simulink model "FlightDynamicModelBlackOut"  (R2017a)
settings: Solver=VariableStepAuto  StartTime=0.0  StopTime=200  RelTol=1e-3
undefined symbols (not defined in the file or in its folder): F, Light, MIL
libraries: simulink x13, aerolibatmos2 x1, aerolibwind2 x1
settings Model: Creator=740582  LastModifiedBy=740582
settings OptimizationCC: LifeSpan=inf
settings DebuggingCC: SFExecutionAtInitializationDiag=none

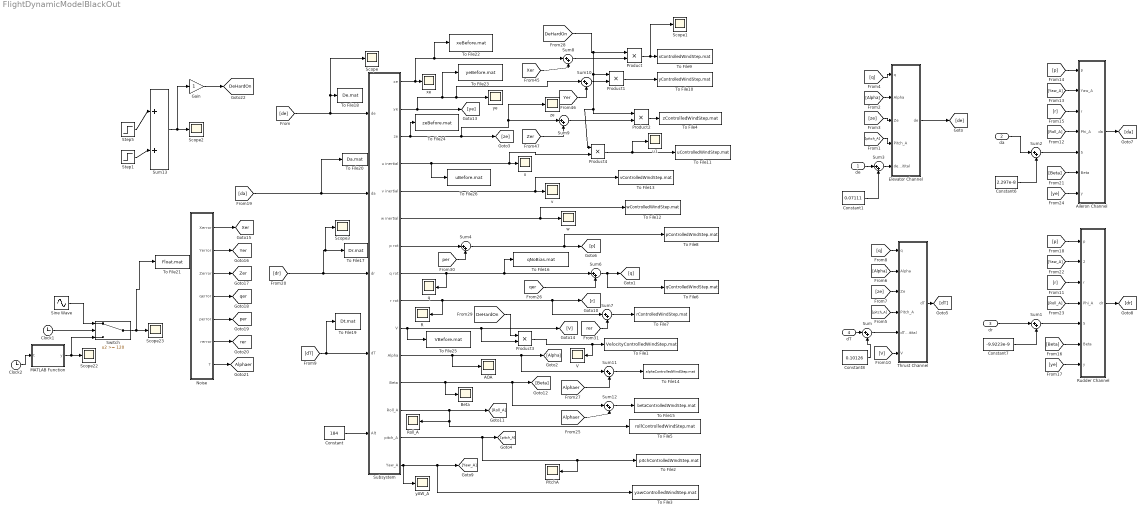
== system FlightDynamicModelBlackOut ==
  de : Inport
  da : Inport  Port=2
  dr : Inport  Port=3
  dT : Inport  Port=4
  AOA : Scope
  Aileron Channel : Subsystem
  "Beta " : Scope
  Clock1 : Clock
  Clock2 : Clock
  Constant : Constant  Value=184
  Constant1 : Constant  Value=0.07111
  Constant6 : Constant  Value=2.297e-8
  Constant7 : Constant  Value=-9.9223e-9
  Constant8 : Constant  Value=0.10126
  Elevator Channel : Subsystem
  Gain : Gain
  MATLAB Function : MATLAB Function  TreatAsAtomicUnit=on
  Noise : Subsystem
  PitchA : Scope
  Product{,1..4} (5 alike) : Product
  "R " : Scope
  "Roll_A " : Scope
  Rudder Channel : Subsystem
  Scope{,1..3,22..23} (6 alike) : Scope
  Sine Wave : Sin  Amplitude=0.1745  Frequency=0.1833  Phase=pi  SampleTime=0
  Step1 : Step  Time=80  SampleTime=20
  Step5 : Step  Time=40  Before=1  After=0  SampleTime=20
  Subsystem : Subsystem
  Sum{,1..4,6..13} (13 alike) : Sum  Inputs=|++
  Switch : Switch  Threshold=120
  Thrust Channel : Subsystem
  To File1 : ToFile  Filename=VelocityControlledWindStep.mat  MatrixName=VelocityControlledWindStep
  To File10 : ToFile  Filename=yControlledWindStep.mat  MatrixName=yControlledWindStep
  To File11 : ToFile  Filename=uControlledWindStep.mat  MatrixName=uControlledWindStep
  To File12 : ToFile  Filename=wControlledWindStep.mat  MatrixName=wControlledWindStep
  To File13 : ToFile  Filename=vControlledWindStep.mat  MatrixName=vControlledWindStep
  To File14 : ToFile  Filename=alphaControlledWindStep.mat  MatrixName=alphaControlledWindStep
  To File15 : ToFile  Filename=betaControlledWindStep.mat  MatrixName=betaControlledWindStep
  To File16 : ToFile  Filename=qNoBias.mat  MatrixName=qNoBias
  To File17 : ToFile  Filename=Dr.mat  MatrixName=Dr
  To File18 : ToFile  Filename=De.mat  MatrixName=De
  To File19 : ToFile  Filename=Dt.mat  MatrixName=Dt
  To File2 : ToFile  Filename=pitchControlledWindStep.mat  MatrixName=pitchControlledWindStep
  To File20 : ToFile  Filename=Da.mat  MatrixName=Da
  To File21 : ToFile  Filename=Float.mat  MatrixName=Float
  To File22 : ToFile  Filename=xeBefore.mat  MatrixName=xeBefore
  To File23 : ToFile  Filename=yeBefore.mat  MatrixName=yeBefore
  To File24 : ToFile  Filename=zeBefore.mat  MatrixName=zeBefore
  To File25 : ToFile  Filename=VBefore.mat  MatrixName=VBefore
  To File26 : ToFile  Filename=uBefore.mat  MatrixName=uBefore
  To File3 : ToFile  Filename=yawControlledWindStep.mat  MatrixName=yawControlledWindStep
  To File4 : ToFile  Filename=zControlledWindStep.mat  MatrixName=zControlledWindStep
  To File5 : ToFile  Filename=rollControlledWindStep.mat  MatrixName=rollControlledWindStep
  To File6 : ToFile  Filename=qControlledWindStep.mat  MatrixName=qControlledWindStep
  To File7 : ToFile  Filename=rControlledWindStep.mat  MatrixName=rControlledWindStep
  To File8 : ToFile  Filename=pControlledWindStep.mat  MatrixName=pControlledWindStep
  To File9 : ToFile  Filename=xControlledWindStep.mat  MatrixName=xControlledWindStep
  V : Scope
  q : Scope
  u : Scope
  u1 : Scope
  v : Scope
  w : Scope
  xe : Scope
  yAW_A : Scope
  ye : Scope
  ze : Scope
  tag scope: Alphaer=global, DeHardOn=global, Xer=global, Yer=global, Zer=global, per=global, qer=global, rer=global
  wires:
  Sum1/1 -> Rudder Channel/5(dr_Initital)
  [ze] -> Thrust Channel/3(Ze)
  [p] -> Rudder Channel/1(p)
  [r] -> Aileron Channel/3(r)
  [Beta] -> Rudder Channel/6(Beta)
  [V] -> Thrust Channel/6(V)
  [p] -> Aileron Channel/1(p)
  [pitch_A] -> Elevator Channel/4(Pitch_A)
  Sum3/1 -> Elevator Channel/5(de_Initital)
  Thrust Channel/1(dT) -> [dT]
  Rudder Channel/1(dr) -> [dr]
  [Roll_A] -> Aileron Channel/4(Phi_A)
  [Beta] -> Aileron Channel/6(Beta)
  [Alpha] -> Elevator Channel/2(Alpha)
  [r] -> Rudder Channel/3(r)
  dT/1 -> Sum/1
  [ze] -> Elevator Channel/3(Ze)
  [ye] -> Aileron Channel/7(y)
  da/1 -> Sum2/1
  Sum2/1 -> Aileron Channel/5(da_Initital)
  [q] -> Elevator Channel/1(q)
  [pitch_A] -> Thrust Channel/4(Pitch_A)
  [Yaw_A] -> Aileron Channel/2(Yaw_A)
  [ye] -> Rudder Channel/7(y)
  [Yaw_A] -> Rudder Channel/2(Yaw_A)
  Aileron Channel/1(da) -> [da]
  de/1 -> Sum3/1
  Elevator Channel/1(de) -> [de]
  [Roll_A] -> Rudder Channel/4(Phi_A)
  [q] -> Thrust Channel/1(q)
  Sum/1 -> Thrust Channel/5(dT_Initital)
  [Alpha] -> Thrust Channel/2(Alpha)
  dr/1 -> Sum1/1
  Subsystem/13(Roll_A) -> To File5/1, "Roll_A "/1, [Roll_A]
  Subsystem/15(Yaw_A) -> yAW_A/1, To File3/1, [Yaw_A]
  Subsystem/14(pitch_A) -> PitchA/1, To File2/1, [pitch_A]
  Subsystem/10(V) -> To File25/1, Product3/2, [V]
  Subsystem/6(w inertial) -> w/1, To File12/1
  Subsystem/5(v inertial) -> To File13/1, v/1
  Constant1/1 -> Sum3/2
  Constant/1 -> Subsystem/5(Alt)
  Constant6/1 -> Sum2/2
  Constant8/1 -> Sum/2
  Constant7/1 -> Sum1/2
  Subsystem/1(xe) -> To File22/1, Sum8/1, xe/1
  Subsystem/3(ze) -> To File24/1, ze/1, Sum9/1, [ze]
  Subsystem/2(ye) -> [ye], To File23/1, Sum10/1, ye/1
  Subsystem/8(q rot) -> q/1, Sum6/1, To File16/1
  Subsystem/4(u inertial) -> To File26/1, Product4/2, u/1
  Subsystem/11(Alpha) -> AOA/1, Sum11/1, [Alpha]
  Subsystem/12(Beta) -> Sum12/1, [Beta], "Beta "/1
  Noise/7(Alphaerror) -> [Alphaer]
  Noise/1(Xerror) -> [Xer]
  Noise/2(Yerror) -> [Yer]
  Noise/3(Zerror) -> [Zer]
  Noise/4(qerror) -> [qer]
  Noise/5(perror) -> [per]
  Noise/6(rerror) -> [rer]
  [rer] -> Sum7/2
  [per] -> Sum4/2
  Sum7/1 -> To File7/1
  Subsystem/9(r rot) -> "R "/1, Sum7/1, [r]
  [Yer] -> Sum10/2
  [Xer] -> Sum8/2
  [Zer] -> Sum9/2
  [Alphaer] -> Sum12/2
  [Alphaer] -> Sum11/2
  Sum11/1 -> To File14/1
  Sum12/1 -> To File15/1
  Subsystem/7(p rot) -> Sum4/1
  Sum4/1 -> To File8/1, [p]
  Sum6/1 -> To File6/1, [q]
  [qer] -> Sum6/2
  [DeHardOn] -> Product/1, Product1/1, Product4/1, Product2/1
  [dT] -> To File19/1, Subsystem/4(dT)
  Switch/1 -> To File21/1, Scope23/1
  Clock1/1 -> Switch/2
  Sine Wave/1 -> Switch/1
  Clock2/1 -> MATLAB Function/1(t)
  MATLAB Function/1(y) -> Scope22/1, Switch/3
  [dr] -> Scope3/1, To File17/1, Subsystem/3(dr)
  [da] -> To File20/1, Subsystem/2(da)
  [de] -> Scope/1, To File18/1, Subsystem/1(de)
  Step1/1 -> Sum13/2
  Step5/1 -> Sum13/1
  Sum13/1 -> Gain/1, Scope2/1
  Sum8/1 -> Product/2
  Product/1 -> Scope1/1, To File9/1
  Sum10/1 -> Product1/2
  Product1/1 -> To File10/1
  Sum9/1 -> Product2/2
  Product2/1 -> To File4/1
  Product3/1 -> V/1, To File1/1
  [DeHardOn] -> Product3/1
  Product4/1 -> u1/1, To File11/1
  Gain/1 -> [DeHardOn]

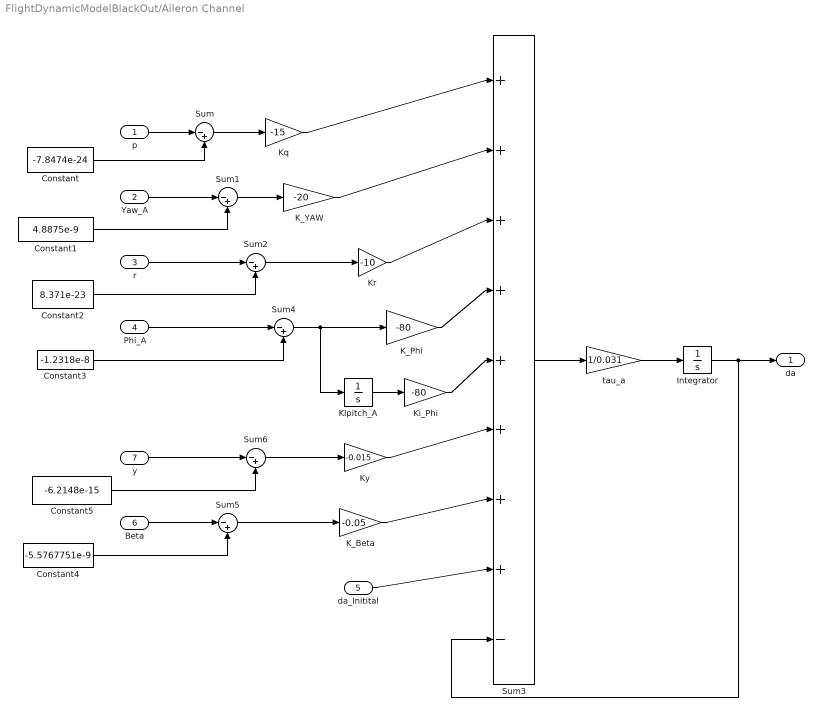
== system FlightDynamicModelBlackOut/Aileron Channel ==
  p : Inport
  Yaw_A : Inport  Port=2
  r : Inport  Port=3
  Phi_A : Inport  Port=4
  da_Initital : Inport  Port=5
  Beta : Inport  Port=6
  y : Inport  Port=7
  Constant : Constant  Value=-7.8474e-24
  Constant1 : Constant  Value=4.8875e-9
  Constant2 : Constant  Value=8.371e-23
  Constant3 : Constant  Value=-1.2318e-8
  Constant4 : Constant  Value=-5.5767751e-9
  Constant5 : Constant  Value=-6.2148e-15
  Integrator : Integrator  InitialCondition=2.297e-8  LimitOutput=on  UpperSaturationLimit=0.3490658504  LowerSaturationLimit=-0.3490658504
  KIpitch_A : Integrator
  K_Beta : Gain  Gain=-0.05
  K_Phi : Gain  Gain=-80
  K_YAW : Gain  Gain=-20
  Ki_Phi : Gain  Gain=-80
  Kq : Gain  Gain=-15
  Kr : Gain  Gain=-10
  Ky : Gain  Gain=-0.015
  Sum{,1..2,4..6} (6 alike) : Sum  Inputs=|-+
  Sum3 : Sum  Inputs=|++++++++-
  tau_a : Gain  Gain=1/0.031
  da : Outport  OutMin=[-0.3490658504]  OutMax=[0.3490658504]
  wires:
  Constant/1 -> Sum/2
  p/1 -> Sum/1
  Yaw_A/1 -> Sum1/1
  r/1 -> Sum2/1
  Phi_A/1 -> Sum4/1
  Constant1/1 -> Sum1/2
  Constant2/1 -> Sum2/2
  Constant3/1 -> Sum4/2
  Sum/1 -> Kq/1
  Sum1/1 -> K_YAW/1
  Sum2/1 -> Kr/1
  Sum4/1 -> KIpitch_A/1, K_Phi/1
  Kq/1 -> Sum3/1
  K_YAW/1 -> Sum3/2
  Kr/1 -> Sum3/3
  K_Phi/1 -> Sum3/4
  Sum3/1 -> tau_a/1
  Ki_Phi/1 -> Sum3/5
  KIpitch_A/1 -> Ki_Phi/1
  tau_a/1 -> Integrator/1
  Integrator/1 -> Sum3/9, da/1
  da_Initital/1 -> Sum3/8
  K_Beta/1 -> Sum3/7
  Beta/1 -> Sum5/1
  Sum5/1 -> K_Beta/1
  Constant4/1 -> Sum5/2
  Ky/1 -> Sum3/6
  y/1 -> Sum6/1
  Sum6/1 -> Ky/1
  Constant5/1 -> Sum6/2

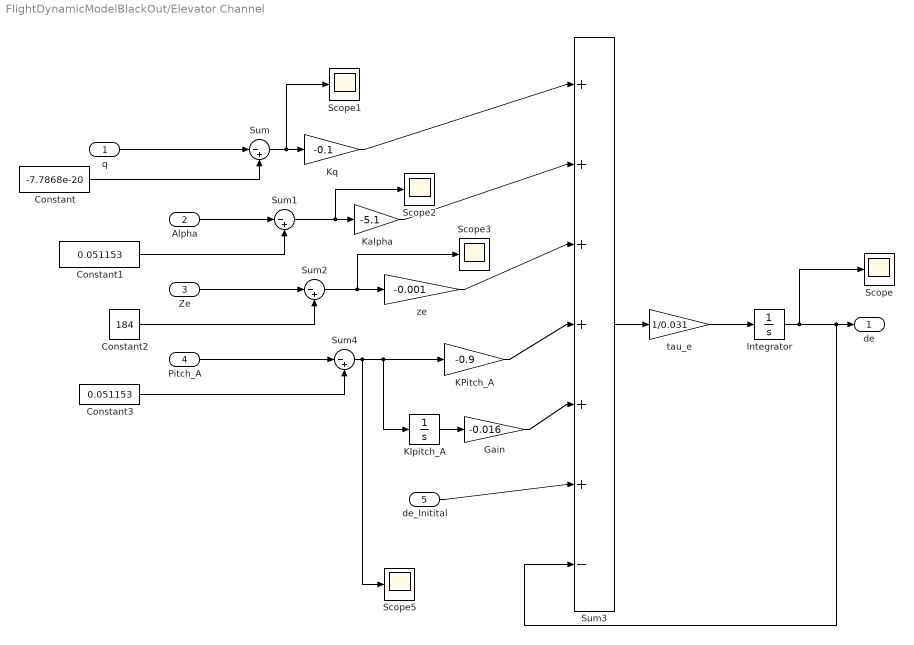
== system FlightDynamicModelBlackOut/Elevator Channel ==
  q : Inport
  Alpha : Inport  Port=2
  Ze : Inport  Port=3
  Pitch_A : Inport  Port=4
  de_Initital : Inport  Port=5
  Constant : Constant  Value=-7.7868e-20
  Constant1 : Constant  Value=0.051153
  Constant2 : Constant  Value=184
  Constant3 : Constant  Value=0.051153
  Gain : Gain  Gain=-0.016
  Integrator : Integrator  InitialCondition=0.07111  LimitOutput=on  UpperSaturationLimit=0.3490658504  LowerSaturationLimit=-0.6981317008
  KIpitch_A : Integrator
  KPitch_A : Gain  Gain=-0.9
  Kalpha : Gain  Gain=-5.1
  Kq : Gain  Gain=-0.1
  Scope{,1..3,5} (5 alike) : Scope
  Sum{,1..2,4} (4 alike) : Sum  Inputs=|-+
  Sum3 : Sum  Inputs=|++++++-
  tau_e : Gain  Gain=1/0.031
  ze : Gain  Gain=-0.001
  de : Outport  OutMin=[-0.6981317008504]  OutMax=[0.3490658504]
  wires:
  Alpha/1 -> Sum1/1
  Ze/1 -> Sum2/1
  Pitch_A/1 -> Sum4/1
  Constant1/1 -> Sum1/2
  Constant2/1 -> Sum2/2
  Constant3/1 -> Sum4/2
  Sum/1 -> Scope1/1, Kq/1
  Sum1/1 -> Scope2/1, Kalpha/1
  Sum2/1 -> Scope3/1, ze/1
  Sum4/1 -> Scope5/1, KIpitch_A/1, KPitch_A/1
  Kq/1 -> Sum3/1
  Kalpha/1 -> Sum3/2
  ze/1 -> Sum3/3
  KPitch_A/1 -> Sum3/4
  Sum3/1 -> tau_e/1
  de_Initital/1 -> Sum3/6
  Gain/1 -> Sum3/5
  KIpitch_A/1 -> Gain/1
  tau_e/1 -> Integrator/1
  Integrator/1 -> Scope/1, Sum3/7, de/1
  q/1 -> Sum/1
  Constant/1 -> Sum/2

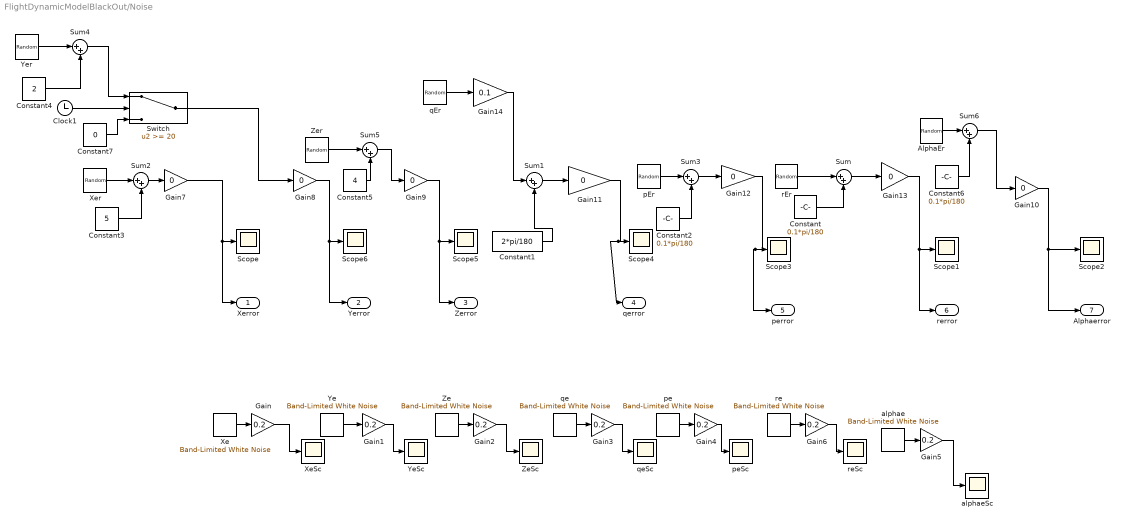
== system FlightDynamicModelBlackOut/Noise ==
  AlphaEr : UniformRandomNumber  Minimum=-0.001*0.1014*pi/180  Maximum=0.001*0.1014*pi/180  SampleTime=0.1
  Clock1 : Clock
  Constant : Constant  Value=0.1*pi/180
  Constant1 : Constant  Value=2*pi/180
  Constant2 : Constant  Value=0.1*pi/180
  Constant3 : Constant  Value=5
  Constant4 : Constant  Value=2
  Constant5 : Constant  Value=4
  Constant6 : Constant  Value=0.1*pi/180
  Constant7 : Constant  Value=0
  Gain{,1..6} (7 alike) : Gain  Gain=0.2
  Gain{7..13} (7 alike) : Gain  Gain=0
  Gain14 : Gain  Gain=0.1
  Scope{,1..6} (7 alike) : Scope
  Sum{,1..6} (7 alike) : Sum  Inputs=|++
  Switch : Switch  Threshold=20
  Xe : simulink/Sources/Band-Limited White Noise  Cov=[0.8]  Ts=0.1  seed=[23341]
  XeSc : Scope
  Xer : UniformRandomNumber  Minimum=-2  Maximum=2  SampleTime=0.1
  Ye : simulink/Sources/Band-Limited White Noise  Cov=[0.1*0.5]  Ts=0.1  seed=[23341]
  YeSc : Scope
  Yer : UniformRandomNumber  Minimum=-0.05  Maximum=0.05  SampleTime=0.1
  Ze : simulink/Sources/Band-Limited White Noise  Cov=[0.1]  Ts=0.1  seed=[23341]
  ZeSc : Scope
  Zer : UniformRandomNumber  SampleTime=0.1
  alphae : simulink/Sources/Band-Limited White Noise  Cov=[0.0000008]  Ts=0.1  seed=[23341]
  alphaeSc : Scope
  pEr : UniformRandomNumber  Minimum=-0.001*1.8707*pi/180  Maximum=0.001*1.8707*pi/180  SampleTime=0.1
  pe : simulink/Sources/Band-Limited White Noise  Cov=[0.0001]  Ts=0.1  seed=[23341]
  peSc : Scope
  qEr : UniformRandomNumber  Minimum=-0.001*1.8707*pi/180  Maximum=0.001*1.8707*pi/180  SampleTime=0.1
  qe : simulink/Sources/Band-Limited White Noise  Cov=[0.0001]  Ts=0.1  seed=[23341]
  qeSc : Scope
  rEr : UniformRandomNumber  Minimum=-0.001*1.8707*pi/180  Maximum=0.001*1.8707*pi/180  SampleTime=0.1
  re : simulink/Sources/Band-Limited White Noise  Cov=[0.0001]  Ts=0.1  seed=[23341]
  reSc : Scope
  Xerror : Outport
  Yerror : Outport  Port=2
  Zerror : Outport  Port=3
  qerror : Outport  Port=4
  perror : Outport  Port=5
  rerror : Outport  Port=6
  Alphaerror : Outport  Port=7
  wires:
  alphae/1 -> Gain5/1
  re/1 -> Gain6/1
  Ze/1 -> Gain2/1
  Ye/1 -> Gain1/1
  pe/1 -> Gain4/1
  Xe/1 -> Gain/1
  qe/1 -> Gain3/1
  Gain/1 -> XeSc/1
  Gain1/1 -> YeSc/1
  Gain2/1 -> ZeSc/1
  Gain3/1 -> qeSc/1
  Gain4/1 -> peSc/1
  Gain6/1 -> reSc/1
  Gain5/1 -> alphaeSc/1
  Gain7/1 -> Xerror/1, Scope/1
  Gain8/1 -> Yerror/1, Scope6/1
  Gain9/1 -> Zerror/1, Scope5/1
  Gain10/1 -> Alphaerror/1, Scope2/1
  Gain13/1 -> rerror/1, Scope1/1
  Gain12/1 -> perror/1, Scope3/1
  Gain11/1 -> qerror/1, Scope4/1
  Sum1/1 -> Gain11/1
  Sum3/1 -> Gain12/1
  pEr/1 -> Sum3/1
  rEr/1 -> Sum/1
  Sum/1 -> Gain13/1
  Sum2/1 -> Gain7/1
  Constant/1 -> Sum/2
  Constant2/1 -> Sum3/2
  Constant1/1 -> Sum1/2
  Xer/1 -> Sum2/1
  Yer/1 -> Sum4/1
  qEr/1 -> Gain14/1
  AlphaEr/1 -> Sum6/1
  Sum6/1 -> Gain10/1
  Constant3/1 -> Sum2/2
  Constant4/1 -> Sum4/2
  Constant6/1 -> Sum6/2
  Constant7/1 -> Switch/3
  Clock1/1 -> Switch/2
  Zer/1 -> Sum5/1
  Sum5/1 -> Gain9/1
  Constant5/1 -> Sum5/2
  Sum4/1 -> Switch/1
  Switch/1 -> Gain8/1
  Gain14/1 -> Sum1/1

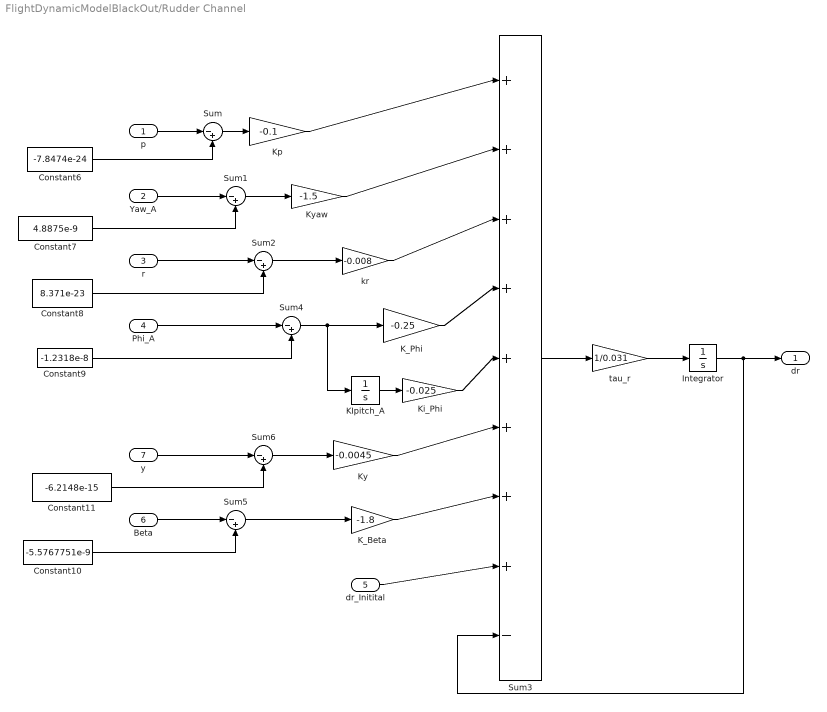
== system FlightDynamicModelBlackOut/Rudder Channel ==
  p : Inport
  Yaw_A : Inport  Port=2
  r : Inport  Port=3
  Phi_A : Inport  Port=4
  dr_Initital : Inport  Port=5
  Beta : Inport  Port=6
  y : Inport  Port=7
  Constant10 : Constant  Value=-5.5767751e-9
  Constant11 : Constant  Value=-6.2148e-15
  Constant6 : Constant  Value=-7.8474e-24
  Constant7 : Constant  Value=4.8875e-9
  Constant8 : Constant  Value=8.371e-23
  Constant9 : Constant  Value=-1.2318e-8
  Integrator : Integrator  InitialCondition=-9.9223e-9  LimitOutput=on  UpperSaturationLimit=0.5235987756  LowerSaturationLimit=-0.5235987756
  KIpitch_A : Integrator
  K_Beta : Gain  Gain=-1.8
  K_Phi : Gain  Gain=-0.25
  Ki_Phi : Gain  Gain=-0.025
  Kp : Gain  Gain=-0.1
  Ky : Gain  Gain=-0.0045
  Kyaw : Gain  Gain=-1.5
  Sum{,1..2,4..6} (6 alike) : Sum  Inputs=|-+
  Sum3 : Sum  Inputs=|++++++++-
  "kr " : Gain  Gain=-0.008
  tau_r : Gain  Gain=1/0.031
  dr : Outport  OutMin=[-0.5235987756]  OutMax=[0.5235987756]
  wires:
  dr_Initital/1 -> Sum3/8
  Sum6/1 -> Ky/1
  y/1 -> Sum6/1
  Beta/1 -> Sum5/1
  Sum5/1 -> K_Beta/1
  Constant10/1 -> Sum5/2
  K_Beta/1 -> Sum3/7
  Phi_A/1 -> Sum4/1
  Constant7/1 -> Sum1/2
  Ki_Phi/1 -> Sum3/5
  Constant11/1 -> Sum6/2
  K_Phi/1 -> Sum3/4
  Constant6/1 -> Sum/2
  Sum1/1 -> Kyaw/1
  Kyaw/1 -> Sum3/2
  KIpitch_A/1 -> Ki_Phi/1
  Yaw_A/1 -> Sum1/1
  Sum/1 -> Kp/1
  "kr "/1 -> Sum3/3
  r/1 -> Sum2/1
  Sum3/1 -> tau_r/1
  Sum2/1 -> "kr "/1
  Integrator/1 -> Sum3/9, dr/1
  Sum4/1 -> K_Phi/1, KIpitch_A/1
  tau_r/1 -> Integrator/1
  Kp/1 -> Sum3/1
  Constant8/1 -> Sum2/2
  Ky/1 -> Sum3/6
  p/1 -> Sum/1
  Constant9/1 -> Sum4/2

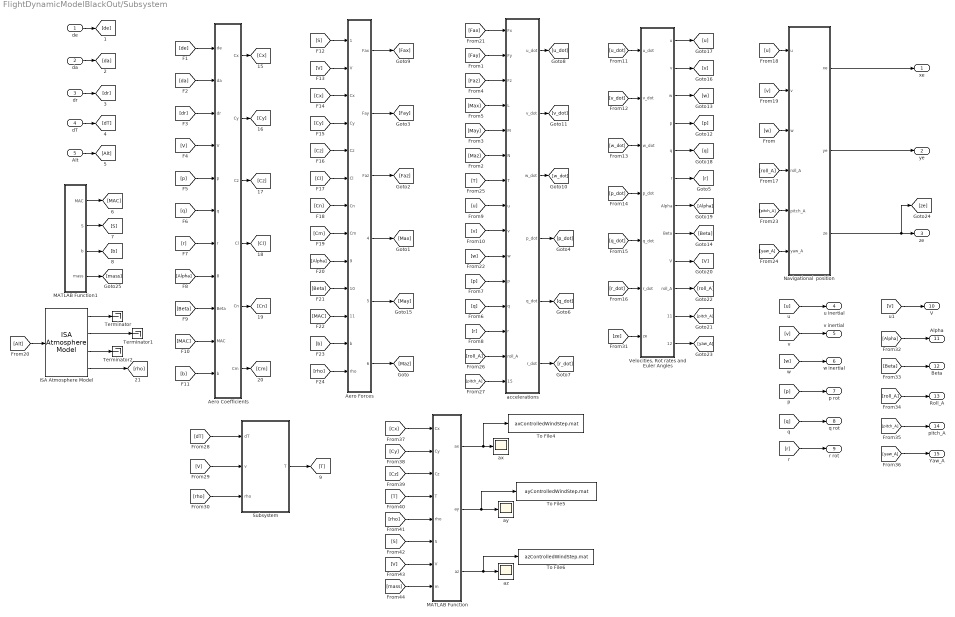
== system FlightDynamicModelBlackOut/Subsystem ==
  de : Inport
  da : Inport  Port=2
  dr : Inport  Port=3
  dT : Inport  Port=4
  Alt : Inport  Port=5
  Aero Coefficients : MATLAB Function  TreatAsAtomicUnit=on
  Aero Forces : MATLAB Function  TreatAsAtomicUnit=on
  ISA Atmosphere Model : aerolibatmos2/ISA Atmosphere Model  custom=off  g=9.80665  gamma=1.4  R=287.0531  L=0.0065  h_trop=11000  h_strat=20000  rho0=1.225  P0=101325  T0=288.15  h0=0
      settings: SourceProductName=Aerospace Blockset
  MATLAB Function : MATLAB Function  TreatAsAtomicUnit=on
  MATLAB Function1 : MATLAB Function  TreatAsAtomicUnit=on
  Navigational  position : Subsystem
  Subsystem : Subsystem
  Terminator : Terminator
  Terminator1 : Terminator
  Terminator2 : Terminator
  To File4 : ToFile  Filename=axControlledWindStep.mat  MatrixName=axControlledWindStep
  To File5 : ToFile  Filename=ayControlledWindStep.mat  MatrixName=ayControlledWindStep
  To File6 : ToFile  Filename=azControlledWindStep.mat  MatrixName=azControlledWindStep
  "Velocities, Rot rates and Euler Angles" : Subsystem
  accelerations : MATLAB Function  TreatAsAtomicUnit=on
  ax : Scope
  ay : Scope
  az : Scope
  xe : Outport
  ye : Outport  Port=2
  ze : Outport  Port=3
  u inertial : Outport  Port=4
  v inertial : Outport  Port=5
  w inertial : Outport  Port=6
  p rot : Outport  Port=7
  q rot : Outport  Port=8
  r rot : Outport  Port=9
  V : Outport  Port=10
  Alpha : Outport  Port=11
  Beta : Outport  Port=12
  Roll_A : Outport  Port=13
  pitch_A : Outport  Port=14
  Yaw_A : Outport  Port=15
  wires:
  de/1 -> [de]
  da/1 -> [da]
  dr/1 -> [dr]
  dT/1 -> [dT]
  Alt/1 -> [Alt]
  MATLAB Function1/1(MAC) -> [MAC]
  MATLAB Function1/2(S) -> [S]
  MATLAB Function1/3(b) -> [b]
  [de] -> Aero Coefficients/1(de)
  [da] -> Aero Coefficients/2(da)
  [dr] -> Aero Coefficients/3(dr)
  [V] -> Aero Coefficients/4(V)
  [b] -> Aero Coefficients/11(b)
  [MAC] -> Aero Coefficients/10(MAC)
  [Beta] -> Aero Coefficients/9(Beta)
  [Alpha] -> Aero Coefficients/8(alpha)
  Aero Coefficients/1(Cx) -> [Cx]
  Aero Coefficients/2(Cy) -> [Cy]
  Aero Coefficients/3(Cz) -> [Cz]
  Aero Coefficients/4(Cl) -> [Cl]
  Aero Coefficients/5(Cn) -> [Cn]
  Aero Coefficients/6(Cm) -> [Cm]
  [Cx] -> Aero Forces/3(Cx)
  [p] -> Aero Coefficients/5(p)
  [q] -> Aero Coefficients/6(q)
  [r] -> Aero Coefficients/7(r)
  [Cy] -> Aero Forces/4(Cy)
  [Cz] -> Aero Forces/5(Cz)
  [Cl] -> Aero Forces/6(Cl)
  [Cn] -> Aero Forces/7(Cn)
  [Cm] -> Aero Forces/8(Cm)
  [Alpha] -> Aero Forces/9(alpha)
  [Beta] -> Aero Forces/10(Beta)
  [MAC] -> Aero Forces/11(MAC)
  [b] -> Aero Forces/12(b)
  [rho] -> Aero Forces/13(rho)
  [V] -> Aero Forces/2(V)
  [S] -> Aero Forces/1(Sref)
  ISA Atmosphere Model/1 -> Terminator/1
  ISA Atmosphere Model/2 -> Terminator1/1
  ISA Atmosphere Model/3 -> Terminator2/1
  ISA Atmosphere Model/4 -> [rho]
  [Alt] -> ISA Atmosphere Model/1
  Aero Forces/1(Fax) -> [Fax]
  Aero Forces/2(Fay) -> [Fay]
  Aero Forces/3(Faz) -> [Faz]
  Aero Forces/4(Max) -> [Max]
  Aero Forces/5(May) -> [May]
  Aero Forces/6(Maz) -> [Maz]
  [Fax] -> accelerations/1(Fx)
  [Fay] -> accelerations/2(Fy)
  [Faz] -> accelerations/3(Fz)
  [Max] -> accelerations/4(L)
  [May] -> accelerations/5(M)
  [Maz] -> accelerations/6(N)
  [u] -> accelerations/8(u)
  [v] -> accelerations/9(v)
  [w] -> accelerations/10(w)
  [p] -> accelerations/11(p)
  [q] -> accelerations/12(q)
  [r] -> accelerations/13(r)
  accelerations/1(u_dot) -> [u_dot]
  accelerations/2(v_dot) -> [v_dot]
  accelerations/3(w_dot) -> [w_dot]
  accelerations/4(p_dot) -> [p_dot]
  accelerations/5(q_dot) -> [q_dot]
  accelerations/6(r_dot) -> [r_dot]
  [u_dot] -> "Velocities, Rot rates and Euler Angles"/1(u_dot)
  [v_dot] -> "Velocities, Rot rates and Euler Angles"/2(v_dot)
  [w_dot] -> "Velocities, Rot rates and Euler Angles"/3(w_dot)
  [p_dot] -> "Velocities, Rot rates and Euler Angles"/4(p_dot)
  [q_dot] -> "Velocities, Rot rates and Euler Angles"/5(q_dot)
  [r_dot] -> "Velocities, Rot rates and Euler Angles"/6(r_dot)
  "Velocities, Rot rates and Euler Angles"/7(Alpha) -> [Alpha]
  "Velocities, Rot rates and Euler Angles"/8(Beta) -> [Beta]
  "Velocities, Rot rates and Euler Angles"/9(V) -> [V]
  "Velocities, Rot rates and Euler Angles"/10(roll_A) -> [roll_A]
  "Velocities, Rot rates and Euler Angles"/11(pitch_A) -> [pitch_A]
  "Velocities, Rot rates and Euler Angles"/12(yaw_A) -> [yaw_A]
  [u] -> Navigational  position/1(u)
  [v] -> Navigational  position/2(v)
  [w] -> Navigational  position/3(w)
  [roll_A] -> Navigational  position/4(roll_A)
  [pitch_A] -> Navigational  position/5(pitch_A)
  [yaw_A] -> Navigational  position/6(yaw_A)
  [u] -> u inertial/1
  [v] -> v inertial/1
  [w] -> w inertial/1
  [p] -> p rot/1
  [q] -> q rot/1
  [r] -> r rot/1
  [V] -> V/1
  [T] -> accelerations/7(T)
  [roll_A] -> accelerations/14(roll_A)
  [pitch_A] -> accelerations/15(pitch_A)
  [dT] -> Subsystem/1(dT)
  [V] -> Subsystem/2(v)
  [rho] -> Subsystem/3(rho)
  Subsystem/1(T) -> [T]
  "Velocities, Rot rates and Euler Angles"/6(r) -> [r]
  "Velocities, Rot rates and Euler Angles"/5(q) -> [q]
  "Velocities, Rot rates and Euler Angles"/4(p) -> [p]
  "Velocities, Rot rates and Euler Angles"/3(w) -> [w]
  "Velocities, Rot rates and Euler Angles"/2(v) -> [v]
  "Velocities, Rot rates and Euler Angles"/1(u) -> [u]
  [ze] -> "Velocities, Rot rates and Euler Angles"/7(ze)
  [Alpha] -> Alpha/1
  [Beta] -> Beta/1
  [roll_A] -> Roll_A/1
  [pitch_A] -> pitch_A/1
  [yaw_A] -> Yaw_A/1
  [mass] -> MATLAB Function/8(m)
  [V] -> MATLAB Function/7(V)
  MATLAB Function/3(az) -> To File6/1, az/1
  MATLAB Function/1(ax) -> To File4/1, ax/1
  [Cy] -> MATLAB Function/2(Cy)
  [T] -> MATLAB Function/4(T)
  [S] -> MATLAB Function/6(S)
  [Cz] -> MATLAB Function/3(Cz)
  MATLAB Function/2(ay) -> To File5/1, ay/1
  [Cx] -> MATLAB Function/1(Cx)
  [rho] -> MATLAB Function/5(rho)
  MATLAB Function1/4(mass) -> [mass]
  Navigational  position/1(xe) -> xe/1
  Navigational  position/2(ye) -> ye/1
  Navigational  position/3(ze) -> [ze], ze/1

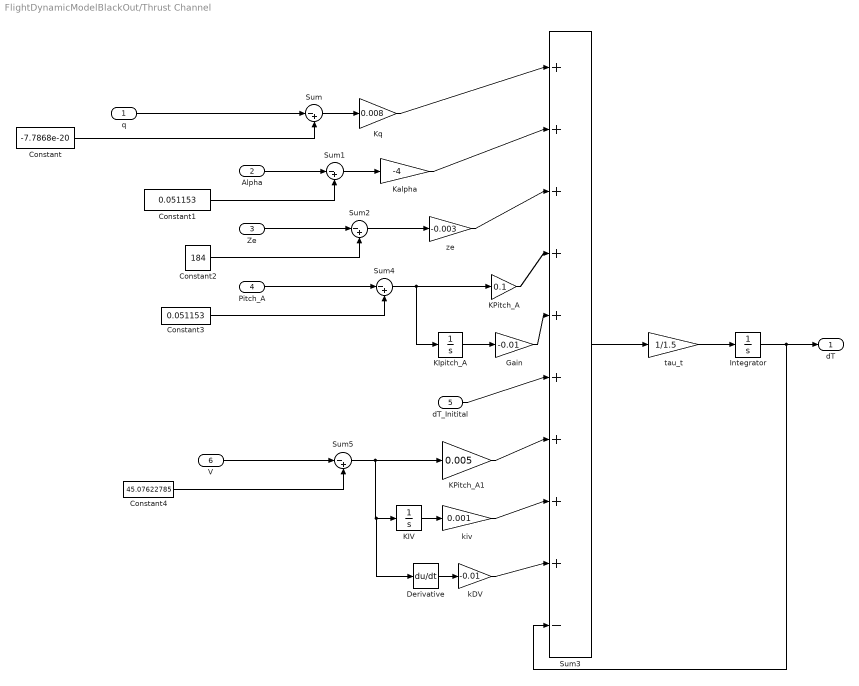
== system FlightDynamicModelBlackOut/Thrust Channel ==
  q : Inport
  Alpha : Inport  Port=2
  Ze : Inport  Port=3
  Pitch_A : Inport  Port=4
  dT_Initital : Inport  Port=5
  V : Inport  Port=6
  Constant : Constant  Value=-7.7868e-20
  Constant1 : Constant  Value=0.051153
  Constant2 : Constant  Value=184
  Constant3 : Constant  Value=0.051153
  Constant4 : Constant  Value=45.07622785
  Derivative : Derivative
  Gain : Gain  Gain=-0.01
  Integrator : Integrator  InitialCondition=0.10126  LimitOutput=on  UpperSaturationLimit=1  LowerSaturationLimit=0
  KIV : Integrator
  KIpitch_A : Integrator
  KPitch_A : Gain  Gain=0.1
  KPitch_A1 : Gain  Gain=0.005
  Kalpha : Gain  Gain=-4
  Kq : Gain  Gain=0.008
  Sum{,1..2,4..5} (5 alike) : Sum  Inputs=|-+
  Sum3 : Sum  Inputs=|+++++++++-
  kDV : Gain  Gain=-0.01
  "kiv " : Gain  Gain=0.001
  tau_t : Gain  Gain=1/1.5
  ze : Gain  Gain=-0.003
  dT : Outport  OutMin=[0]  OutMax=[1]
  wires:
  Alpha/1 -> Sum1/1
  Ze/1 -> Sum2/1
  Pitch_A/1 -> Sum4/1
  Constant1/1 -> Sum1/2
  Constant2/1 -> Sum2/2
  Constant3/1 -> Sum4/2
  Sum/1 -> Kq/1
  Sum1/1 -> Kalpha/1
  Sum2/1 -> ze/1
  Sum4/1 -> KPitch_A/1, KIpitch_A/1
  Kq/1 -> Sum3/1
  Kalpha/1 -> Sum3/2
  ze/1 -> Sum3/3
  KPitch_A/1 -> Sum3/4
  Sum3/1 -> tau_t/1
  dT_Initital/1 -> Sum3/6
  Gain/1 -> Sum3/5
  KIpitch_A/1 -> Gain/1
  tau_t/1 -> Integrator/1
  Integrator/1 -> Sum3/10, dT/1
  KPitch_A1/1 -> Sum3/7
  KIV/1 -> "kiv "/1
  Constant4/1 -> Sum5/2
  Sum5/1 -> Derivative/1, KIV/1, KPitch_A1/1
  V/1 -> Sum5/1
  "kiv "/1 -> Sum3/8
  kDV/1 -> Sum3/9
  Derivative/1 -> kDV/1
  q/1 -> Sum/1
  Constant/1 -> Sum/2

== system FlightDynamicModelBlackOut/Subsystem/Navigational  position ==
  u : Inport
  v : Inport  Port=2
  w : Inport  Port=3
  roll_A : Inport  Port=4
  pitch_A : Inport  Port=5
  yaw_A : Inport  Port=6
  MATLAB Function : MATLAB Function  TreatAsAtomicUnit=on
  "xe " : Integrator  ContinuousStateAttributes='xPosition'
  "ye " : Integrator  InitialCondition=-6.2148e-15  ContinuousStateAttributes='yPosition'
  "ze " : Integrator  InitialCondition=184  ContinuousStateAttributes='zPosition'
  xe : Outport
  ye : Outport  Port=2
  ze : Outport  Port=3
  wires:
  pitch_A/1 -> MATLAB Function/5(pitch_A)
  yaw_A/1 -> MATLAB Function/6(yaw_A)
  roll_A/1 -> MATLAB Function/4(roll_A)
  w/1 -> MATLAB Function/3(w)
  v/1 -> MATLAB Function/2(v)
  u/1 -> MATLAB Function/1(u)
  MATLAB Function/1(x_e_dot) -> "xe "/1
  MATLAB Function/2(y_e_dot) -> "ye "/1
  MATLAB Function/3(z_e_dot) -> "ze "/1
  "ze "/1 -> ze/1
  "ye "/1 -> ye/1
  "xe "/1 -> xe/1

== system FlightDynamicModelBlackOut/Subsystem/Subsystem ==
  dT : Inport
  v : Inport  Port=2
  rho : Inport  Port=3
  MATLAB Function : MATLAB Function  TreatAsAtomicUnit=on
  T : Outport
  wires:
  dT/1 -> MATLAB Function/1(dT)
  v/1 -> MATLAB Function/2(V)
  rho/1 -> MATLAB Function/3(rho)
  MATLAB Function/1(T) -> T/1

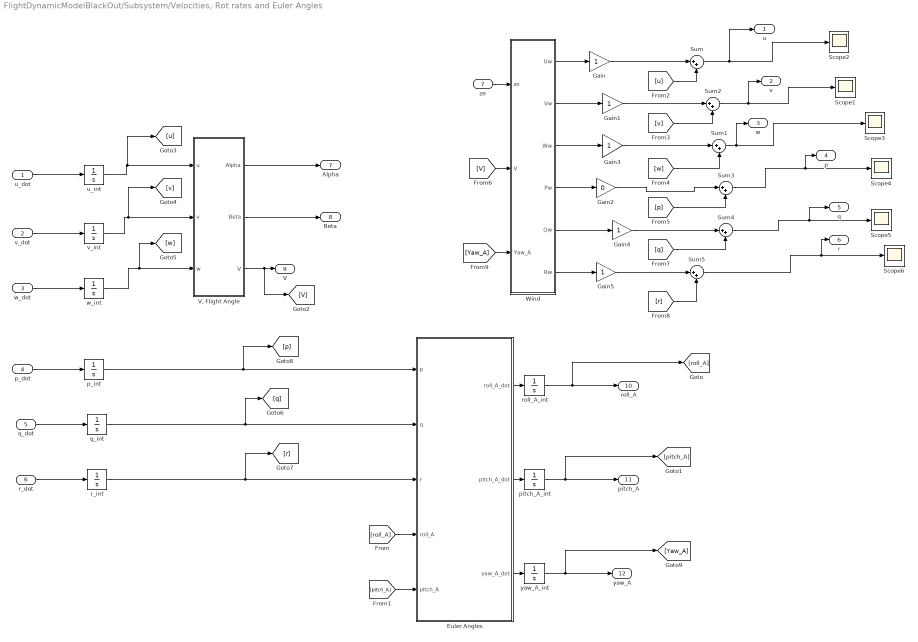
== system FlightDynamicModelBlackOut/Subsystem/Velocities, Rot rates and Euler Angles ==
  u_dot : Inport
  v_dot : Inport  Port=2
  w_dot : Inport  Port=3
  p_dot : Inport  Port=4
  q_dot : Inport  Port=5
  r_dot : Inport  Port=6
  ze : Inport  Port=7
  Euler Angles : MATLAB Function  TreatAsAtomicUnit=on
  Gain{,1,3..5} (5 alike) : Gain
  Gain2 : Gain  Gain=0
  Scope{1..6} (6 alike) : Scope
  Sum{,1..5} (6 alike) : Sum  Inputs=|++
  "V, Flight Angle" : MATLAB Function  TreatAsAtomicUnit=on
  Wind : Subsystem
  p_int : Integrator  InitialCondition=-7.8474e-24  ContinuousStateAttributes='velocity_p'
  pitch_A_int : Integrator  InitialCondition=0.051153  ContinuousStateAttributes='pitch_A'
  q_int : Integrator  InitialCondition=-7.7868e-20  ContinuousStateAttributes='velocity_q'
  r_int : Integrator  InitialCondition=8.371e-23  ContinuousStateAttributes='velocity_r'
  roll_A_int : Integrator  InitialCondition=-1.22318e-8  ContinuousStateAttributes='roll_A'
  u_int : Integrator  InitialCondition=45.0151  ContinuousStateAttributes='velocity_u'
  v_int : Integrator  InitialCondition=-2.4869e-7  ContinuousStateAttributes='velocity_v'
  w_int : Integrator  InitialCondition=2.3047  ContinuousStateAttributes='velocity_w'
  yaw_A_int : Integrator  InitialCondition=4.8875e-9  ContinuousStateAttributes='Yaw_A'
  u : Outport
  v : Outport  Port=2
  w : Outport  Port=3
  p : Outport  Port=4
  q : Outport  Port=5
  r : Outport  Port=6
  Alpha : Outport  Port=7
  Beta : Outport  Port=8
  V : Outport  Port=9
  roll_A : Outport  Port=10
  pitch_A : Outport  Port=11
  yaw_A : Outport  Port=12
  wires:
  u_dot/1 -> u_int/1
  u_int/1 -> [u], "V, Flight Angle"/1(u)
  v_dot/1 -> v_int/1
  w_dot/1 -> w_int/1
  p_dot/1 -> p_int/1
  q_dot/1 -> q_int/1
  r_dot/1 -> r_int/1
  v_int/1 -> [v], "V, Flight Angle"/2(v)
  w_int/1 -> [w], "V, Flight Angle"/3(w)
  "V, Flight Angle"/3(V) -> [V], V/1
  Euler Angles/1(roll_A_dot) -> roll_A_int/1
  Euler Angles/2(pitch_A_dot) -> pitch_A_int/1
  Euler Angles/3(yaw_A_dot) -> yaw_A_int/1
  pitch_A_int/1 -> pitch_A/1, [pitch_A]
  roll_A_int/1 -> roll_A/1, [roll_A]
  [roll_A] -> Euler Angles/4(roll_A)
  [pitch_A] -> Euler Angles/5(pitch_A)
  [w] -> Sum1/2
  Wind/5(Qw) -> Gain4/1
  Wind/2("Vw ") -> Gain1/1
  Wind/1("Uw ") -> Gain/1
  Sum4/1 -> q/1, Scope5/1
  [r] -> Sum5/2
  Wind/3("Ww ") -> Gain3/1
  [v] -> Sum2/2
  [q] -> Sum4/2
  Wind/6(Rw) -> Gain5/1
  Sum3/1 -> p/1, Scope4/1
  [p] -> Sum3/2
  Sum1/1 -> w/1, Scope3/1
  Wind/4(Pw) -> Gain2/1
  [V] -> Wind/2(V)
  Sum/1 -> u/1, Scope2/1
  [u] -> Sum/2
  Sum2/1 -> v/1, Scope1/1
  yaw_A_int/1 -> [Yaw_A], yaw_A/1
  [Yaw_A] -> Wind/3(Yaw_A)
  Gain/1 -> Sum/1
  Gain1/1 -> Sum2/1
  Gain3/1 -> Sum1/1
  Gain2/1 -> Sum3/1
  Gain4/1 -> Sum4/1
  Gain5/1 -> Sum5/1
  ze/1 -> Wind/1(ze)
  Sum5/1 -> r/1, Scope6/1
  p_int/1 -> [p], Euler Angles/1(p)
  q_int/1 -> [q], Euler Angles/2(q)
  r_int/1 -> [r], Euler Angles/3(r)
  "V, Flight Angle"/1(Alpha) -> Alpha/1
  "V, Flight Angle"/2(Beta) -> Beta/1

== system FlightDynamicModelBlackOut/Subsystem/Velocities, Rot rates and Euler Angles/Wind ==
  ze : Inport
  V : Inport  Port=2
  Yaw_A : Inport  Port=3
  Constant2 : Constant  Value=2.08751424
  MATLAB Function : MATLAB Function  TreatAsAtomicUnit=on
  "Pw " : Scope
  "Qw " : Scope
  "Rw " : Scope
  Subsystem : Subsystem
  Sum : Sum  Inputs=|++
  Sum1 : Sum  Inputs=|++
  Uw : Scope
  Vw : Scope
  Ww : Scope
  "Uw " : Outport
  "Vw " : Outport  Port=2
  "Ww " : Outport  Port=3
  Pw : Outport  Port=4
  Qw : Outport  Port=5
  Rw : Outport  Port=6
  wires:
  V/1 -> Subsystem/2(V)
  Subsystem/6(Rw) -> Rw/1, "Rw "/1
  Subsystem/3(Ww) -> Ww/1, "Ww "/1
  ze/1 -> Subsystem/1(h), [ze]
  Constant2/1 -> Subsystem/3(b)
  Subsystem/4(Pw) -> Pw/1, "Pw "/1
  Subsystem/5(Qw) -> Qw/1, "Qw "/1
  [ze] -> MATLAB Function/1(ze)
  MATLAB Function/1(uw) -> [uw]
  MATLAB Function/2(vw) -> [vw]
  Yaw_A/1 -> MATLAB Function/2(Yaw_A)
  Subsystem/1(Uw) -> Sum/1
  [uw] -> Sum/2
  Sum/1 -> "Uw "/1, Uw/1
  Subsystem/2(Vw) -> Sum1/1
  [vw] -> Sum1/2
  Sum1/1 -> "Vw "/1, Vw/1

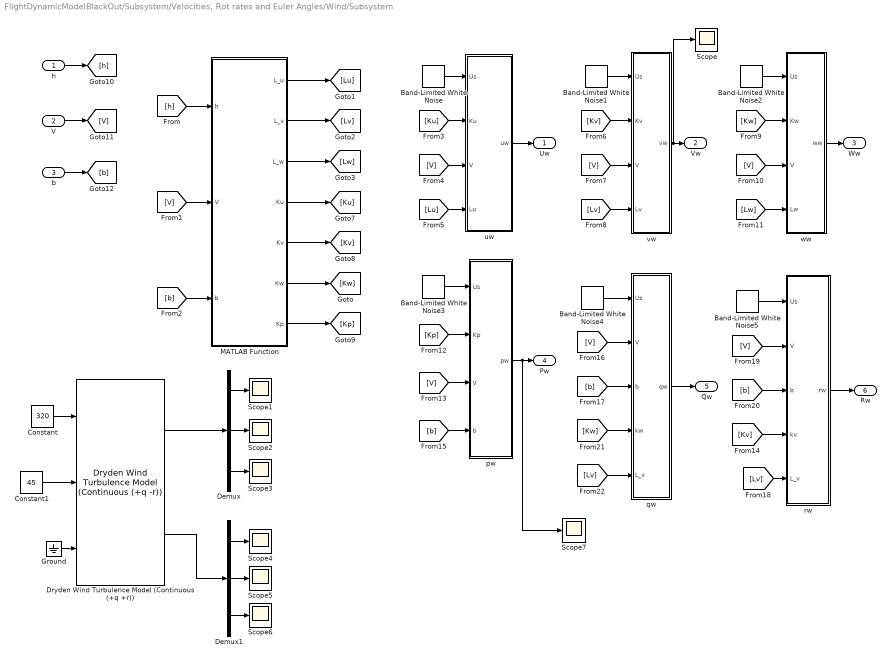
== system FlightDynamicModelBlackOut/Subsystem/Velocities, Rot rates and Euler Angles/Wind/Subsystem ==
  h : Inport
  V : Inport  Port=2
  b : Inport  Port=3
  Band-Limited White Noise : simulink/Sources/Band-Limited White Noise  Cov=[0.0055]  Ts=0.1  seed=[23341]
  Band-Limited White Noise1 : simulink/Sources/Band-Limited White Noise  Cov=[0.0055]  Ts=0.1  seed=[23342]
  Band-Limited White Noise2 : simulink/Sources/Band-Limited White Noise  Cov=[0.0055]  Ts=0.1  seed=[23343]
  Band-Limited White Noise3 : simulink/Sources/Band-Limited White Noise  Cov=[0.000055]  Ts=0.1  seed=[23344]
  Band-Limited White Noise4 : simulink/Sources/Band-Limited White Noise  Cov=[0.000055]  Ts=0.1  seed=[23345]
  Band-Limited White Noise5 : simulink/Sources/Band-Limited White Noise  Cov=[0.000055]  Ts=0.1  seed=[23346]
  Constant : Constant  Value=320
  Constant1 : Constant  Value=45
  Demux : Demux  Outputs=3
  Demux1 : Demux  Outputs=3
  Dryden Wind Turbulence Model (Continuous (+q +r)) : aerolibwind2/Dryden Wind Turbulence Model  (Continuous (+q -r))  units=Metric (MKS)  spec=MIL-F-8785C  model=Continuous Dryden (+q +r)  W20=15  Wdeg=0  TurbProb=10^-2 - Light  L_high=533.4  Wingspan=2.08751424  ts=0.1  Seed=[23341 23342 23343 23344]  T_on=on
      settings: SourceProductName=Aerospace Blockset
  Ground : Ground
  MATLAB Function : MATLAB Function  TreatAsAtomicUnit=on
  Scope{,1..7} (8 alike) : Scope
  pw : Subsystem
  qw : Subsystem
  rw : Subsystem
  uw : Subsystem
  vw : Subsystem
  ww : Subsystem
  Uw : Outport
  Vw : Outport  Port=2
  Ww : Outport  Port=3
  Pw : Outport  Port=4
  Qw : Outport  Port=5
  Rw : Outport  Port=6
  wires:
  MATLAB Function/1(L_u) -> [Lu]
  MATLAB Function/2(L_v) -> [Lv]
  MATLAB Function/3(L_w) -> [Lw]
  MATLAB Function/5(Kv) -> [Kv]
  MATLAB Function/6(Kw) -> [Kw]
  MATLAB Function/7(Kp) -> [Kp]
  h/1 -> [h]
  V/1 -> [V]
  b/1 -> [b]
  [h] -> MATLAB Function/1(h)
  [b] -> MATLAB Function/3(b)
  [V] -> MATLAB Function/2(V)
  Band-Limited White Noise/1 -> uw/1(Us)
  [Ku] -> uw/2(Ku)
  [V] -> uw/3(V)
  [Lu] -> uw/4(Lu)
  vw/1(vw) -> Scope/1, Vw/1
  uw/1(uw) -> Uw/1
  Band-Limited White Noise1/1 -> vw/1(Us)
  [Kv] -> vw/2(Kv)
  [V] -> vw/3(V)
  [Lv] -> vw/4(Lv)
  ww/1(ww) -> Ww/1
  Band-Limited White Noise2/1 -> ww/1(Us)
  [Kw] -> ww/2(Kw)
  [V] -> ww/3(V)
  [Lw] -> ww/4(Lw)
  Band-Limited White Noise3/1 -> pw/1(Us)
  [Kp] -> pw/2(Kp)
  [V] -> pw/3(V)
  [b] -> pw/4(b)
  [V] -> qw/2(V)
  [b] -> qw/3(b)
  qw/1(qw) -> Qw/1
  [b] -> rw/3(b)
  [V] -> rw/2(V)
  Band-Limited White Noise5/1 -> rw/1(Us)
  rw/1(rw) -> Rw/1
  MATLAB Function/4(Ku) -> [Ku]
  [Kv] -> rw/4(kv)
  [Lv] -> rw/5(L_v)
  Band-Limited White Noise4/1 -> qw/1(Us)
  [Kw] -> qw/4(kw)
  [Lv] -> qw/5(L_v)
  Constant/1 -> Dryden Wind Turbulence Model (Continuous (+q +r))/1
  Constant1/1 -> Dryden Wind Turbulence Model (Continuous (+q +r))/2
  Ground/1 -> Dryden Wind Turbulence Model (Continuous (+q +r))/3
  Dryden Wind Turbulence Model (Continuous (+q +r))/1 -> Demux/1
  Dryden Wind Turbulence Model (Continuous (+q +r))/2 -> Demux1/1
  Demux/1 -> Scope1/1
  Demux/2 -> Scope2/1
  Demux/3 -> Scope3/1
  Demux1/3 -> Scope6/1
  Demux1/2 -> Scope5/1
  Demux1/1 -> Scope4/1
  pw/1(pw) -> Pw/1, Scope7/1

== system FlightDynamicModelBlackOut/Subsystem/Velocities, Rot rates and Euler Angles/Wind/Subsystem/pw ==
  Us : Inport
  Kp : Inport  Port=2
  V : Inport  Port=3
  b : Inport  Port=4
  MATLAB Function : MATLAB Function  TreatAsAtomicUnit=on
  Product : Product
  Product1 : Product
  Product2 : Product
  Sum : Sum  Inputs=|+-
  pwInt : Integrator
  pw : Outport
  wires:
  Kp/1 -> Product/2
  Us/1 -> Product/1
  Product/1 -> Sum/1
  Sum/1 -> pwInt/1  "sV(s)"
  Product1/1 -> Sum/2
  MATLAB Function/1(k) -> [Con]
  [Con] -> Product1/2
  b/1 -> MATLAB Function/2(b)
  V/1 -> MATLAB Function/1(V)
  Product2/1 -> pw/1
  pwInt/1 -> Product2/2, Product1/1  "Vs"
  [Con] -> Product2/1

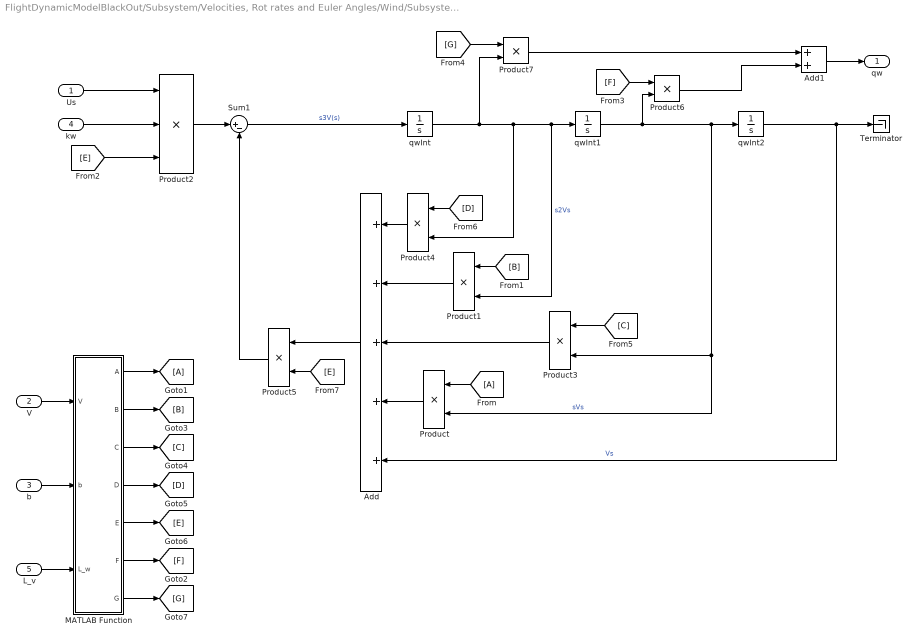
== system FlightDynamicModelBlackOut/Subsystem/Velocities, Rot rates and Euler Angles/Wind/Subsystem/qw ==
  Us : Inport
  V : Inport  Port=2
  b : Inport  Port=3
  kw : Inport  Port=4
  L_v : Inport  Port=5
  Add : Sum  Inputs=+++++
  Add1 : Sum
  MATLAB Function : MATLAB Function  TreatAsAtomicUnit=on
  Product{,1,3..7} (7 alike) : Product
  Product2 : Product  Inputs=3
  Sum1 : Sum  Inputs=|+-
  Terminator : Terminator
  qwInt : Integrator
  qwInt1 : Integrator
  qwInt2 : Integrator
  qw : Outport
  wires:
  MATLAB Function/2(B) -> [B]
  Product3/1 -> Add/3
  [C] -> Product3/1
  Product4/1 -> Add/1
  Add/1 -> Product5/1
  [E] -> Product2/3
  [D] -> Product4/1
  kw/1 -> Product2/2
  [F] -> Product6/1
  [A] -> Product/1
  Product7/1 -> Add1/1
  [G] -> Product7/1
  MATLAB Function/3(C) -> [C]
  Add1/1 -> qw/1
  [E] -> Product5/2
  L_v/1 -> MATLAB Function/3(L_w)
  MATLAB Function/4(D) -> [D]
  qwInt/1 -> Product4/2, Product1/2, qwInt1/1, Product7/2  "s2Vs"
  Product/1 -> Add/4
  [B] -> Product1/1
  MATLAB Function/7(G) -> [G]
  Product6/1 -> Add1/2
  Product5/1 -> Sum1/2
  Us/1 -> Product2/1
  MATLAB Function/1(A) -> [A]
  Product2/1 -> Sum1/1
  qwInt1/1 -> Product6/2, Product3/2, Product/2, qwInt2/1  "sVs"
  MATLAB Function/6(F) -> [F]
  V/1 -> MATLAB Function/1(V)
  b/1 -> MATLAB Function/2(b)
  Product1/1 -> Add/2
  MATLAB Function/5(E) -> [E]
  qwInt2/1 -> Terminator/1, Add/5  "Vs"
  Sum1/1 -> qwInt/1  "s3V(s)"

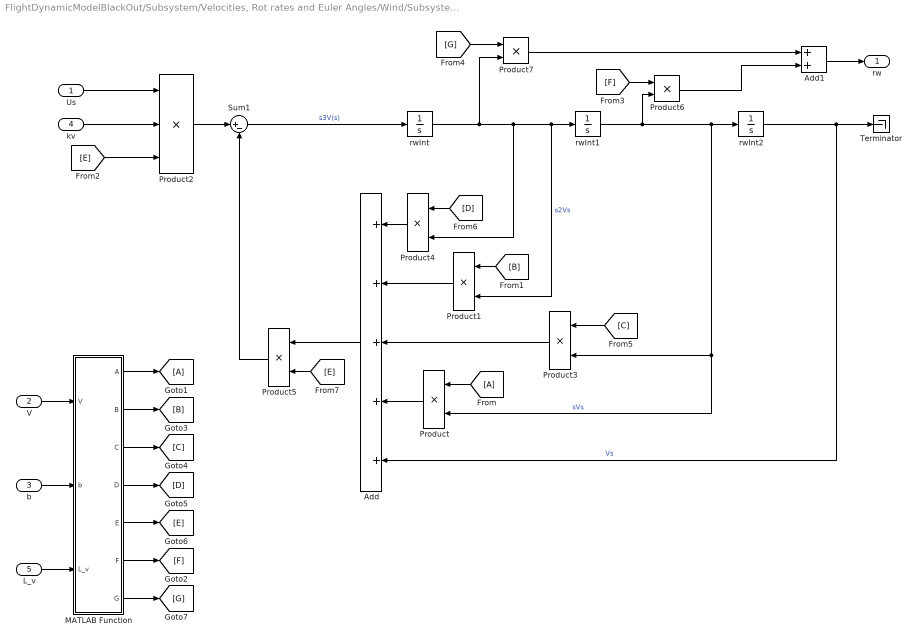
== system FlightDynamicModelBlackOut/Subsystem/Velocities, Rot rates and Euler Angles/Wind/Subsystem/rw ==
  Us : Inport
  V : Inport  Port=2
  b : Inport  Port=3
  kv : Inport  Port=4
  L_v : Inport  Port=5
  Add : Sum  Inputs=+++++
  Add1 : Sum
  MATLAB Function : MATLAB Function  TreatAsAtomicUnit=on
  Product{,1,3..7} (7 alike) : Product
  Product2 : Product  Inputs=3
  Sum1 : Sum  Inputs=|+-
  Terminator : Terminator
  rwInt : Integrator
  rwInt1 : Integrator
  rwInt2 : Integrator
  rw : Outport
  wires:
  Us/1 -> Product2/1
  MATLAB Function/1(A) -> [A]
  Product2/1 -> Sum1/1
  b/1 -> MATLAB Function/2(b)
  V/1 -> MATLAB Function/1(V)
  Sum1/1 -> rwInt/1  "s3V(s)"
  kv/1 -> Product2/2
  MATLAB Function/2(B) -> [B]
  MATLAB Function/3(C) -> [C]
  MATLAB Function/4(D) -> [D]
  MATLAB Function/5(E) -> [E]
  rwInt/1 -> Product4/2, Product1/2, rwInt1/1, Product7/2  "s2Vs"
  rwInt1/1 -> Product6/2, Product3/2, Product/2, rwInt2/1  "sVs"
  rwInt2/1 -> Terminator/1, Add/5  "Vs"
  Product/1 -> Add/4
  [A] -> Product/1
  Product1/1 -> Add/2
  [B] -> Product1/1
  Product3/1 -> Add/3
  [C] -> Product3/1
  Product4/1 -> Add/1
  Add/1 -> Product5/1
  Product5/1 -> Sum1/2
  [E] -> Product5/2
  [E] -> Product2/3
  [D] -> Product4/1
  L_v/1 -> MATLAB Function/3(L_v)
  MATLAB Function/6(F) -> [F]
  MATLAB Function/7(G) -> [G]
  [F] -> Product6/1
  [G] -> Product7/1
  Product6/1 -> Add1/2
  Product7/1 -> Add1/1
  Add1/1 -> rw/1

== system FlightDynamicModelBlackOut/Subsystem/Velocities, Rot rates and Euler Angles/Wind/Subsystem/uw ==
  Us : Inport
  Ku : Inport  Port=2
  V : Inport  Port=3
  Lu : Inport  Port=4
  Product : Product  Inputs=3
  Product1 : Product
  Product2 : Product  Inputs=*/
  Sum : Sum  Inputs=|+-
  uwInt : Integrator
  uw : Outport
  wires:
  Ku/1 -> Product/2
  Us/1 -> Product/1
  Product/1 -> Sum/1
  uwInt/1 -> Sum/2, uw/1  "Vs"
  V/1 -> Product2/1
  Lu/1 -> Product2/2
  Product2/1 -> [Con]
  [Con] -> Product/3
  Sum/1 -> Product1/2
  [Con] -> Product1/1
  Product1/1 -> uwInt/1  "sV(s)"

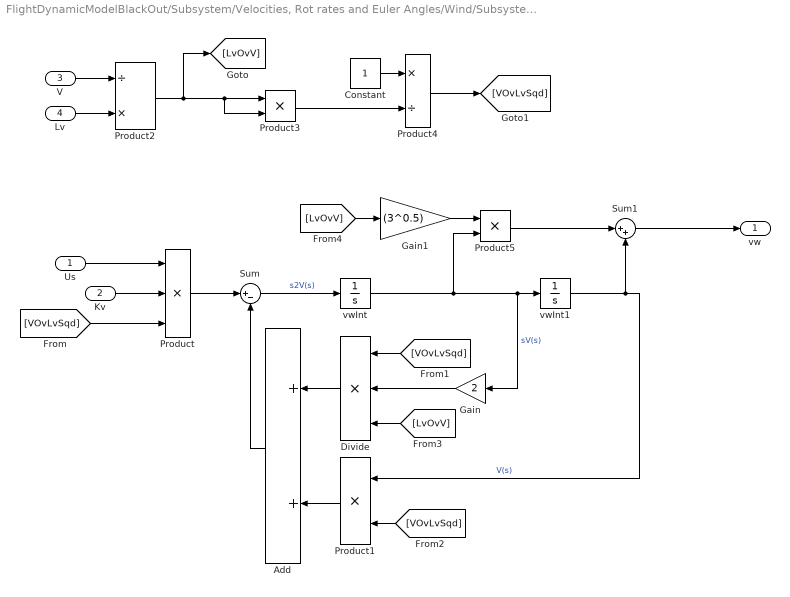
== system FlightDynamicModelBlackOut/Subsystem/Velocities, Rot rates and Euler Angles/Wind/Subsystem/vw ==
  Us : Inport
  Kv : Inport  Port=2
  V : Inport  Port=3
  Lv : Inport  Port=4
  Add : Sum
  Constant : Constant
  Divide : Product  Inputs=***
  Gain : Gain  Gain=2
  Gain1 : Gain  Gain=(3^0.5)
  Product : Product  Inputs=3
  Product1 : Product
  Product2 : Product  Inputs=/*
  Product3 : Product
  Product4 : Product  Inputs=*/
  Product5 : Product
  Sum : Sum  Inputs=|+-
  Sum1 : Sum  Inputs=|++
  vwInt : Integrator
  vwInt1 : Integrator
  vw : Outport
  wires:
  Kv/1 -> Product/2
  Us/1 -> Product/1
  Lv/1 -> Product2/2
  V/1 -> Product2/1
  Product2/1 -> Product3/2, Product3/1, [LvOvV]
  Product3/1 -> Product4/2
  Constant/1 -> Product4/1
  Product4/1 -> [VOvLvSqd]
  [VOvLvSqd] -> Product/3
  Product/1 -> Sum/1
  Sum/1 -> vwInt/1  "s2V(s)"
  vwInt/1 -> Product5/2, Gain/1, vwInt1/1  "sV(s)"
  vwInt1/1 -> Product1/1, Sum1/2  "V(s)"
  Add/1 -> Sum/2
  Divide/1 -> Add/1
  [VOvLvSqd] -> Divide/1
  Gain/1 -> Divide/2
  [LvOvV] -> Divide/3
  Product1/1 -> Add/2
  [VOvLvSqd] -> Product1/2
  Sum1/1 -> vw/1
  Product5/1 -> Sum1/1
  Gain1/1 -> Product5/1
  [LvOvV] -> Gain1/1

== system FlightDynamicModelBlackOut/Subsystem/Velocities, Rot rates and Euler Angles/Wind/Subsystem/ww ==
  Us : Inport
  Kw : Inport  Port=2
  V : Inport  Port=3
  Lw : Inport  Port=4
  Add : Sum
  Constant : Constant
  Divide : Product  Inputs=***
  Gain : Gain  Gain=2
  Gain1 : Gain  Gain=(3^0.5)
  Product : Product  Inputs=3
  Product1 : Product
  Product2 : Product  Inputs=/*
  Product3 : Product
  Product4 : Product  Inputs=*/
  Product5 : Product
  Sum : Sum  Inputs=|+-
  Sum1 : Sum  Inputs=|++
  wwInt : Integrator
  wwInt2 : Integrator
  ww : Outport
  wires:
  Kw/1 -> Product/2
  Lw/1 -> Product2/2
  V/1 -> Product2/1
  Product2/1 -> Product3/2, Product3/1, [LwOvV]
  Product3/1 -> Product4/2
  Constant/1 -> Product4/1
  Product4/1 -> [VOvLwSqd]
  [VOvLwSqd] -> Product/3
  Product/1 -> Sum/1
  Sum/1 -> wwInt/1  "s2V(s)"
  wwInt/1 -> Product5/2, Gain/1, wwInt2/1  "sV(s)"
  wwInt2/1 -> Product1/1, Sum1/2  "V(s)"
  Add/1 -> Sum/2
  Divide/1 -> Add/1
  [VOvLwSqd] -> Divide/1
  Gain/1 -> Divide/2
  [LwOvV] -> Divide/3
  Product1/1 -> Add/2
  [VOvLwSqd] -> Product1/2
  Sum1/1 -> ww/1
  Product5/1 -> Sum1/1
  Gain1/1 -> Product5/1
  [LwOvV] -> Gain1/1
  Us/1 -> Product/1

== matlab function FlightDynamicModelBlackOut/Subsystem/MATLAB Function1 ==
  data: MAC output; S output; b output; mass output
function [MAC, S, b, mass] = fcn()
MAC =0.27898344 ;
S = 0.548295;
b =2.08751424;
mass = 22.497960865;


end

== matlab function FlightDynamicModelBlackOut/Subsystem/Aero Coefficients ==
  data: de input; Cx output; da input; dr input; V input; p input; q input; r input; alpha input; Beta input; MAC input; b input; Cy output; Cz output; Cl output; Cn output; Cm output
function [Cx,Cy,Cz,Cl,Cn,Cm] = fcn(de,da,dr,V,p,q,r,alpha,Beta,MAC,b)
%For Cx
A = -0.0390905 + (0.35218*alpha) + (5.36708*alpha^2) -(23.1537*alpha^3) - (26.2264*alpha^4) + (109.938*alpha^5);
B = ((q*(2.46995+(24.4028*alpha)+(58.4581*alpha^2))*MAC)/(2*V)) + (0.125409*alpha*de) + (0.0857469*alpha^3*de) - (0.00961977*alpha^5*de);
C = -0.0811392*de^2 + (0.0405696*alpha^2*de^2) - (0.0033808*alpha^4*de^2)-(0.389796*alpha*de^3)+ (0.064966*alpha^3*de^3) - 0.0032483*alpha^5*de^3;
%For Cy_______________________________________________________________

D = (-1.0499*Beta) + (0.254159*Beta^3) + ((b*r*(0.765433+0.10909*alpha+0.553414*alpha^2))/(2*V));
E = (b*p*((1.22326*alpha)+(1.26322*alpha^2)- (39.4599*alpha^3))/(2*V)) + (0.175591*dr);

%For Cz________________________________________________________________

F =  -0.0261857 - (5.38662*alpha) + (0.339087*alpha^2) + (28.0138*alpha^3) - (23.0418*alpha^4) - (12.8899*alpha^5);
G = (MAC*q*(-28.2259-(62.5918*alpha) - (460.841*alpha^2))/(2*V)) - (0.445354*de) - (de*0.0972682*alpha^2) + (de*0.0347678*alpha^4);
H = (-0.0811392*alpha*de^2) + (0.0135232*alpha^3*de^2) - (0.00067616*alpha^5*de^2) + (0.389796*de^3) - (0.194898*alpha^2*de^3) + (0.0162415*alpha^4*de^3) ;

%For Cl_________________________________________________________________

J = (-0.126318*Beta) - (0.22119*alpha*Beta) + (0.255338*Beta^3) - (0.191268*Beta^5) + (b*r*(0.0608527 + (0.730792*alpha)+ (2.90179*alpha^2))/(2*V)) ;
K = (b*p*(-0.414849 - 0.325859*alpha + (6.67529*alpha^2) + (125.613*alpha^4))/(2*V)) - (0.0247139*da) + (0.0193176*dr);

%For Cm_________________________________________________________________

L =  0.181738 - (1.10553*alpha) - (15.1134*alpha^4) + (MAC*q*(-47.6756 + (69.4945*alpha)+(308.277*alpha^2))/(2*V));
M = (-1.76253*de) - (0.920542*alpha*de^2) +1.35544*de^3  ; 

%For Cn_________________________________________________________________

N =  (0.202546*Beta) - (0.143331*Beta^3) + (b*r*(-0.379639 - (0.205145*alpha) - (0.937344*alpha^2))/(2*V)) ; 
P = (b*p*(-0.00731187-(0.45033*alpha) + (0.724553*alpha^2) + (16.4433*alpha^3))/(2*V)) - (0.112626*dr) - (0.000470559*Beta*dr); 

%Force Coefficients
Cx = A + B + C;
Cy = D + E;
Cz = F + G + H;

%Moment Coefficients
Cl = J + K;
Cm = L + M ;
Cn = N  + P;

end

== matlab function FlightDynamicModelBlackOut/Subsystem/Aero Forces ==
  data: Sref input; Fax output; V input; Cx input; Cy input; Cz input; Cl input; Cn input; Cm input; alpha input; Beta input; MAC input; b input; rho input; Fay output; Faz output; Max output; May output; Maz output
function [Fax, Fay, Faz, Max, May, Maz] = fcn(Sref,V,Cx,Cy,Cz,Cl,Cn,Cm,alpha,Beta, MAC,b ,rho)
%Dynamic Pressure
q_bar= 0.5*rho*Sref*(V^2);

Fax = q_bar*Cx;
Fay = q_bar*Cy;
Faz = q_bar*Cz;

Max = b*q_bar*Cl;
May = MAC*q_bar*Cm;
Maz = b*q_bar*Cn ;

end

== matlab function FlightDynamicModelBlackOut/Subsystem/accelerations ==
  data: Fx input; Fy input; Fz input; L input; M input; N input; T input; u input; u_dot output; v input; w input; p input; q input; r input; v_dot output; w_dot output; p_dot output; q_dot output; r_dot output; roll_A input; pitch_A input
function [u_dot,v_dot,w_dot,p_dot,q_dot,r_dot] = fcn(Fx,Fy,Fz,L,M,N,T,u,v,w,p,q,r, roll_A, pitch_A)
g =9.81 ;
Mass = 22.497960865;
Ixx = 1.79917041965;
Izz = 7.3946310993;
Ixz = 0.162698154;
Iyy = 5.7676495593;

u_dot = (-(Mass*g*sin(pitch_A)) + T - Fx + (Mass*(r*v - q*w)))/Mass;
v_dot = ((Mass*g*cos(pitch_A)*sin(roll_A)) + Fy + (Mass*(p*w - r*u)))/Mass;
w_dot = ((Mass*g*cos(pitch_A)*cos(roll_A)) + Fz + (Mass*(q*u - p*v)))/Mass;

delta = Ixx*Izz -Ixz^2;

r_dot  = (Ixx*(N - (Ixz*q*r) + ((Ixx-Iyy)*p*q))/delta) + (Ixz*(L + (Ixz*q*p) + (Iyy - Izz)*q*r)/delta);
p_dot = (Izz*(L + (Ixz*p*q) + (Iyy -Izz)*q*r)/delta) + (Ixz*(N - Ixz*q*r +(Ixx-Iyy)*p*q)/delta);
q_dot = (1/Iyy)*(M - ((Ixx-Izz)*p*r) - (Ixz*(p^2 -r^2)));

% A  =  q*r*(Izz - Iyy)- (Ixz*p*q);
% B = (r*p*(Ixx - Izz)) + (Ixz*(p^2 - r^2));
% C = (p*q*(Iyy - Ixx)) + Ixz*q*r;
% D =  Ixx - (Ixz^2)/Izz ;
% 
% p_dot = (L -A + (Ixz/Izz)*(N -C))/D ; 
% q_dot = (M - B)/Iyy;
% r_dot  = (N + Ixz*p_dot -C)/ Izz;

end

== matlab function FlightDynamicModelBlackOut/Subsystem/Velocities, Rot rates and Euler Angles/V, Flight Angle ==
  data: u input; Alpha output; v input; w input; Beta output; V output
function [Alpha,Beta,V] = fcn(u,v,w)

V = (u^2 + v^2 + w^2)^0.5; 
Alpha = atan (w/u);
Beta = asin (v/V);

end

== matlab function FlightDynamicModelBlackOut/Subsystem/Velocities, Rot rates and Euler Angles/Euler Angles ==
  data: p input; roll_A_dot output; q input; r input; roll_A input; pitch_A input; pitch_A_dot output; yaw_A_dot output
function [roll_A_dot, pitch_A_dot,yaw_A_dot] = fcn(p,q,r,roll_A, pitch_A)

roll_A_dot= p + (q*sin(roll_A)*tan(pitch_A)) + (r*cos(roll_A)*tan(pitch_A));
pitch_A_dot= (q*cos(roll_A)) - (r*sin(roll_A));
yaw_A_dot = ((q*sin(roll_A)) + (r*cos(roll_A)))*sec(pitch_A);

end

== matlab function FlightDynamicModelBlackOut/Subsystem/Navigational  position/MATLAB Function ==
  data: u input; x_e_dot output; v input; w input; roll_A input; pitch_A input; yaw_A input; y_e_dot output; z_e_dot output
function [x_e_dot, y_e_dot, z_e_dot] = fcn(u,v,w,roll_A, pitch_A, yaw_A)

x_e_dot = (u*cos(pitch_A)*cos(yaw_A)) + (v*((sin(roll_A)*sin(pitch_A)*cos(yaw_A)) - (cos(roll_A)*sin(roll_A))))+ (w*((cos(roll_A)*sin(pitch_A)*cos(yaw_A)) + (sin(roll_A)*sin(yaw_A))));
y_e_dot = (u*cos(pitch_A)*sin(yaw_A)) + (v*((sin(roll_A)*sin(pitch_A)*sin(yaw_A)) + (cos(roll_A)*cos(roll_A)))) + (w*((cos(roll_A)*sin(pitch_A)*sin(yaw_A)) - (sin(roll_A)*cos(yaw_A))));
z_e_dot = -u*sin(pitch_A) + (v*sin(roll_A)*cos(pitch_A)) + (w*(cos(roll_A)*cos(pitch_A)));

end

== matlab function FlightDynamicModelBlackOut/Subsystem/Subsystem/MATLAB Function ==
  data: dT input; T output; V input; rho input
function T = fcn(dT,V,rho)
%#codegen
K =  0.055;
A = -2.338;
B = 574;
C = 65260;
rho_o = 1.225;
densityFactor = 0.6708669355;

Vlarge = V/((K)^0.5);
Tlarge = ((rho/rho_o)^0.7)*((A*Vlarge^2) +(B*Vlarge) + C)*(dT);
T_one = (Tlarge* K^3)/densityFactor;
T = T_one*2;
end

== matlab function FlightDynamicModelBlackOut/Subsystem/Velocities, Rot rates and Euler Angles/Wind/Subsystem/MATLAB Function ==
  data: h input; L_u output; V input; L_v output; L_w output; b input; Ku output; Kv output; Kw output; Kp output
function [L_u,L_v,L_w,Ku ,Kv ,Kw ,Kp ] = fcn(h,V,b)
%#codegen
%U20= 7.71667;  
%U20= 15.4333;  %moderate
U20 = 23.15;   %severe
%U20 = 0;   %severe
b = 2.08751424;

if h <= 304.8;
Sigma_w = 0.1*U20;
Sigma_u = Sigma_w*(1/(0.177 + 0.000823*h)^0.4);
Sigma_v = Sigma_u;
L_u = h*(1/(0.177 + 0.000823*h)^1.2);
L_v = h*(1/(0.177 + 0.000823*h)^1.2);
L_w = h;

elseif 304.8 < h && h <= 609,6;
        
Sigma_w_lower = 0.1*U20;
Sigma_u_lower = Sigma_w_lower*(1/(0.177 + 0.000823*304.8)^0.4);

Sigma_w_upper = 5;
Sigma_u_upper = Sigma_w_upper;

SigmaGrad_u = (Sigma_u_upper - Sigma_u_lower)/(533.4 -304.8);
SigmaGrad_other = (Sigma_w_upper - Sigma_w_lower)/(533.4 -304.8);
Sigma_w = SigmaGrad_other*(h - 304.8) + Sigma_w_lower ;
Sigma_u = SigmaGrad_u*(h - 304.8) + Sigma_u_upper;
Sigma_v = Sigma_u;
    
L_u_lower = 304.8*(1/(0.177 + 0.000823*304.8)^1.2);
L_w_lower = 304.8;
L_u_upper = 533.4;
L_w_upper = 533.4;
Grad_u = (L_u_upper - L_u_lower)/(533.4 -304.8);
Grad_other = (L_w_upper - L_w_lower)/(533.4 -304.8);
L_u = Grad_u*(h - 304.8) + L_u_lower ;
%L_u = abs(L_u);
L_v = L_u ;
L_w = Grad_other*(h - 304.8) + L_w_lower;

else 
Sigma_w = 5;
Sigma_u = Sigma_w;
Sigma_v = Sigma_u;
L_u = 533.4;
L_v = 533.4;
L_w = 533.4;
end
L_u = abs(L_u);
L_v = L_u;
Ku = Sigma_u *(2*L_u/(pi*V))^0.5 ; 
Kv = Sigma_v *(L_v/(pi*V))^0.5 ;
Kw = Sigma_w *(L_w/(pi*V))^0.5 ;
Kp = Sigma_w *(sqrt(0.8/V))*((1/L_w)^(1/3))*((pi/4*b)^(1/6)) ;

end

== matlab function FlightDynamicModelBlackOut/Subsystem/Velocities, Rot rates and Euler Angles/Wind/Subsystem/pw/MATLAB Function ==
  data: V input; k output; b input
function k = fcn(V,b)
%#codegen

k = pi*V/(4*b) ;
end

== matlab function FlightDynamicModelBlackOut/Subsystem/Velocities, Rot rates and Euler Angles/Wind/Subsystem/qw/MATLAB Function ==
  data: V input; A output; b input; L_w input; B output; C output; D output; E output; F output; G output
function [A, B, C, D, E, F, G ] = fcn(V,b,L_w)
%#codegen
A = (2*L_w)/V;
B = ((L_w)^2)/(V)^2;
C = (4*b)/(pi*V);
D = (8*b*L_w)/(pi*V^2);
E = (pi*V^3)/(4*b*L_w^2);
F = 1/V;
G = (L_w*3^0.5)/V^2 ;
end

== matlab function FlightDynamicModelBlackOut/Subsystem/Velocities, Rot rates and Euler Angles/Wind/Subsystem/rw/MATLAB Function ==
  data: V input; A output; b input; L_v input; B output; C output; D output; E output; F output; G output
function [A, B, C, D, E, F, G ] = fcn(V,b,L_v)
%#codegen
A = (2*L_v)/V;
B = ((L_v)^2)/(V)^2;
C = (3*b)/(pi*V);
D = (6*b*L_v)/(pi*V^2);
E = (pi*V^3 )/(3*b*L_v^2);
F = 1/V;
G = (L_v*3^0.5)/V^2 ;
end

== matlab function FlightDynamicModelBlackOut/Subsystem/Velocities, Rot rates and Euler Angles/Wind/MATLAB Function ==
  data: ze input; uw output; Yaw_A input; vw output
function [uw ,vw] = fcn(ze, Yaw_A)
Vw_Ninem = 0;
%Vw_Ninem= 7.71667;  
Psi_Wind = 0; 

if ze <300
Vw = Vw_Ninem *(ze^0.2545  - 0.4097)/1.347;

else 
Vw = 2.86585*Vw_Ninem;
end

uw = Vw*cos(Psi_Wind - pi)*cos(Yaw_A) + Vw*sin(Psi_Wind - pi)*sin(Yaw_A);
vw = -Vw*cos(Psi_Wind - pi)*sin(Yaw_A) + Vw*sin(Psi_Wind - pi)*cos(Yaw_A);

end

== matlab function FlightDynamicModelBlackOut/Subsystem/MATLAB Function ==
  data: Cx input; ax output; Cy input; Cz input; T input; rho input; S input; V input; m input; ay output; az output
function [ax,ay,az] = fcn(Cx, Cy, Cz, T, rho, S, V, m)
%#codegen
g = 9.81;
ax = (T -(0.5*S*rho*Cx*V^2))/(m);
ay = (0.5*rho*S*Cy*V^2)/m ;
az = (0.5*rho*S*Cz*V^2)/m ;
end

== matlab function FlightDynamicModelBlackOut/MATLAB Function ==
  data: y output; t input
function y = fcn(t)
% Define a time axis:

% Define the period

period = 30;
% Make a function for how the amplitude varies with time:
% For example the amplitude is the square root of time, 
% or whatever formula you want to use.
amplitude = sqrt(t);
% Now make the sine wave
y = amplitude .* sin(2 * pi * t / period)*pi/180;

end
